simulink model "second"  (R2016a)
settings: Solver=VariableStepAuto  StartTime=0.0  StopTime=10.0  RelTol=1e-3
settings Model: Creator=kypis  LastModifiedBy=kypis

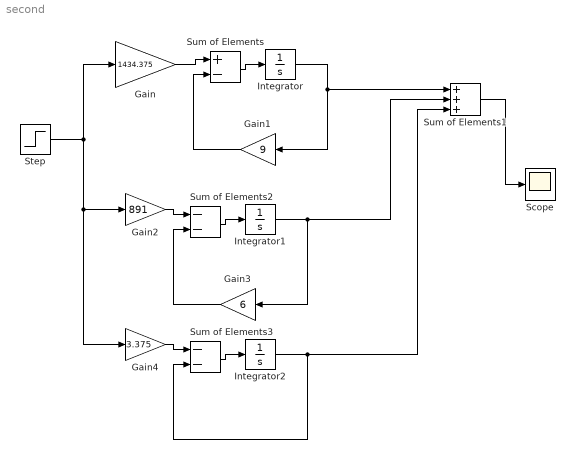
== system second ==
  Gain : Gain  Gain=1434.375
  Gain1 : Gain  Gain=9
  Gain2 : Gain  Gain=891
  Gain3 : Gain  Gain=6
  Gain4 : Gain  Gain=3.375
  Integrator : Integrator
  Integrator1 : Integrator
  Integrator2 : Integrator
  Scope : Scope
  Step : Step  Time=0  SampleTime=0
  Sum of Elements : Sum  Inputs=+-
  Sum of Elements1 : Sum  Inputs=+++
  Sum of Elements2 : Sum  Inputs=--
  Sum of Elements3 : Sum  Inputs=--
  wires:
  Gain/1 -> Sum of Elements/1
  Sum of Elements/1 -> Integrator/1
  Integrator/1 -> Gain1/1, Sum of Elements1/1
  Gain1/1 -> Sum of Elements/2
  Sum of Elements1/1 -> Scope/1
  Gain2/1 -> Sum of Elements2/1
  Sum of Elements2/1 -> Integrator1/1
  Integrator1/1 -> Gain3/1, Sum of Elements1/2
  Gain3/1 -> Sum of Elements2/2
  Step/1 -> Gain4/1, Gain2/1, Gain/1
  Gain4/1 -> Sum of Elements3/1
  Sum of Elements3/1 -> Integrator2/1
  Integrator2/1 -> Sum of Elements3/2, Sum of Elements1/3
